simulink model "simulacion_motor_step_vin_vout"  (R2015b)
settings: Solver=FixedStepAuto  StartTime=0.0  StopTime=1.1  FixedStep=0.00001  RelTol=1e-5
settings Model: Creator=alumno  LastModifiedBy=nico
settings DataIOCC: SaveFormat=Array  SignalLoggingSaveFormat=ModelDataLogs
settings OptimizationCC: ExpressionDepthLimit=2147483647  InitFltsAndDblsToZero=on
settings DebuggingCC: UnderspecifiedInitializationDetection=Classic  MergeDetectMultiDrivingBlocksExec=none  SolverPrmCheckMsg=warning  FcnCallInpInsideContextMsg=UseLocalSettings  StateNameClashWarn=warning
settings HardwareCC: ProdBitPerPointer=32  ProdLargestAtomicFloat=None  ProdIntDivRoundTo=Undefined  ProdEndianess=Unspecified  ProdWordSize=32  ProdHWDeviceType=32-bit Generic
settings GRTTargetCC: CombineOutputUpdateFcns=off  GRTInterface=on
settings ConfigComp: CovModelRefEnable=Off

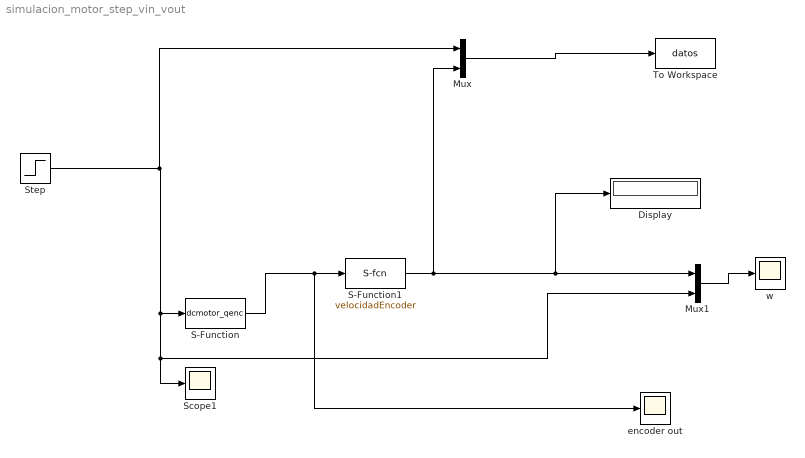
== system simulacion_motor_step_vin_vout ==
  Display : Display
  Mux : Mux  Inputs=2
  Mux1 : Mux  Inputs=2
  S-Function : S-Function  FunctionName=dcmotor_qenc  Parameters=1  SFunctionDeploymentMode=off  EnableBusSupport=off
  S-Function1 : S-Function  FunctionName=velocidadEncoder  Parameters=1 0.00001  SFunctionDeploymentMode=off  EnableBusSupport=off
  Scope1 : Scope
  Step : Step  Time=0.5  After=12  SampleTime=0
  To Workspace : ToWorkspace  VariableName=datos  SaveFormat=Timeseries  SampleTime=-1
  encoder out : Scope
  w : Scope
  wires:
  S-Function/1 -> encoder out/1, S-Function1/1
  Step/1 -> Mux/1, Mux1/2, Scope1/1, S-Function/1
  Mux/1 -> To Workspace/1
  Mux1/1 -> w/1
  S-Function1/1 -> Display/1, Mux1/1, Mux/2
